simulink model "Mech_473_Projectreport_open_loop"  (R2017a)
settings: Solver=VariableStepAuto  StartTime=0.0  StopTime=1  RelTol=1e-3
values from neighbouring files (symbols this model uses):
  JM = 0.00026; sim('Mech473Simp'); plot(t,omega)    [boobies.m]
settings Model: Creator=ni_daly  LastModifiedBy=al_per

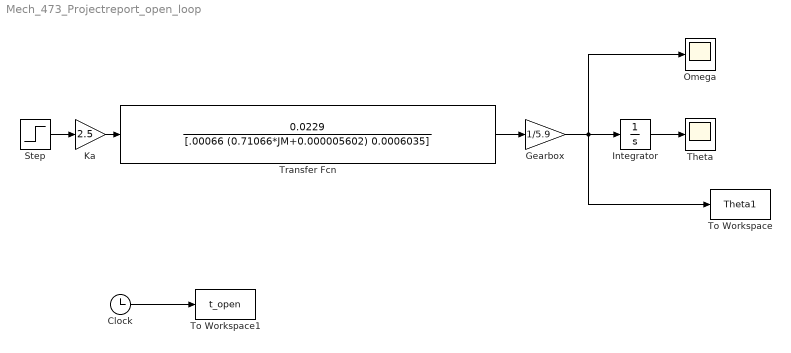
== system Mech_473_Projectreport_open_loop ==
  Clock : Clock
  Gearbox : Gain  Gain=1/5.9
  Integrator : Integrator
  Ka : Gain  Gain=2.5
  Omega : Scope
  Step : Step  Time=0.1  SampleTime=0
  Theta : Scope
  To Workspace : ToWorkspace  VariableName=Theta1  SampleTime=-1
  To Workspace1 : ToWorkspace  VariableName=t_open  SampleTime=-1
  Transfer Fcn : TransferFcn  Numerator=[0.0229]  Denominator=[.00066 (0.71066*JM+0.000005602) 0.0006035]
  wires:
  Integrator/1 -> Theta/1
  Transfer Fcn/1 -> Gearbox/1
  Clock/1 -> To Workspace1/1
  Step/1 -> Ka/1
  Ka/1 -> Transfer Fcn/1
  Gearbox/1 -> To Workspace/1, Omega/1, Integrator/1
